simulink model "heating_plant_reference"  (R2025b)
settings: Solver=FixedStepAuto  StartTime=0.0  StopTime=6000  FixedStep=10  RelTol=1e-3
values from neighbouring files (symbols this model uses):
  K = 40    [run_simulation.m]
  T = 1200    [run_simulation.m]
  Theta_0 = 5    [run_simulation.m]
settings Model: Creator=Thomas  LastModifiedBy=Thomas
settings DataIOCC: SaveOutput=off  SaveTime=off
settings ModelReferenceCC: ModelReferenceMinAlgLoopOccurrences=on

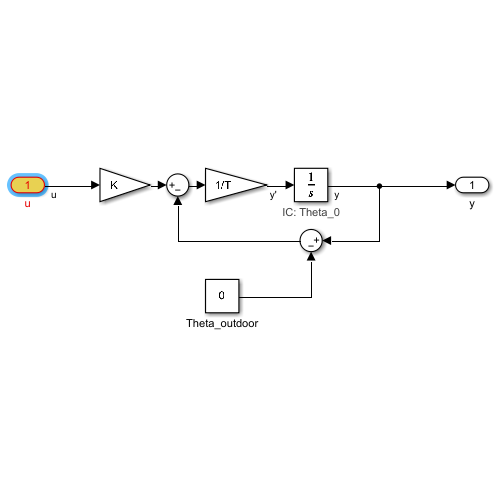
[thumbnail: Simulink's stored preview of the top-level diagram]
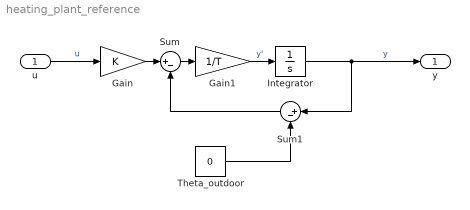
== system heating_plant_reference ==
  u : Inport  OutDataTypeStr=double  PortDimensions=1
  Gain : Gain  Gain=K
  Gain1 : Gain  Gain=1/T
  Integrator : Integrator  InitialCondition=Theta_0
      settings: AttributesFormatString=IC: %<InitialCondition>
  Sum : Sum  Inputs=|+-
  Sum1 : Sum  Inputs=|+-
  Theta_outdoor : Constant  Value=0
  y : Outport  OutDataTypeStr=double  PortDimensions=1  SampleTime=0
  wires:
  Gain1/1 -> Integrator/1  "y'"
  Integrator/1 -> Sum1/1, y/1  "y"
  u/1 -> Gain/1  "u"
  Gain/1 -> Sum/1
  Sum/1 -> Gain1/1
  Sum1/1 -> Sum/2
  Theta_outdoor/1 -> Sum1/2
